simulink model "Simulation_6DOFTesting"  (R2024a)
settings: Solver=ode4  StartTime=initial_time  StopTime=final_time  FixedStep=timestep  RelTol=1e-3
values from neighbouring files (symbols this model uses):
  aEarth = 0    [CodeTesting_6DOF.m]    (also in Constants_6DOF.m = 6378137; Constants_6DOFTesting.m = 6378137)
  alphaArray = [-30, -25, -20, -15, -10, -5, 0, 5, 10, 15, 20, 25, 30]    [CodeTesting_6DOF.m]    (also in Constants_6DOF.m; Constants_6DOFTesting.m)
  altitudeArray = [0, 1000, 2000, 3000, 4000, 5000, 6000, 7000, 8000, 9000, 10000, 15000, 20000,      25000, 30000, 35000, 40000, 45000, 50000, 55000, 60000]    [CodeTesting_6DOF.m]    (also in Constants_6DOF.m; Constants_6DOFTesting.m)
  bEarth = 0    [CodeTesting_6DOF.m]    (also in Constants_6DOF.m = 6356752.3; Constants_6DOFTesting.m = 6356752.3)
  cD_3DArray = zeros(numAoAs, numMachs, numAltitudes)    [CodeTesting_6DOF.m]    (also in Constants_6DOF.m; Constants_6DOFTesting.m)
  cL_3DArray = zeros(numAoAs, numMachs, numAltitudes)    [CodeTesting_6DOF.m]    (also in Constants_6DOF.m; Constants_6DOFTesting.m)
  densityList = rhoList    [CodeTesting_6DOF.m]    (also in Constants_6DOF.m = usAtmosphere.x_; Constants_6DOFTesting.m = usAtmosphere.x_)
  height0 = 0    [Constants_6DOF.m]    (also in Constants_6DOFTesting.m = 5000)
  heightsList = usAtmosphere.Z    [CodeTesting_6DOF.m]    (also in Constants_6DOF.m; Constants_6DOFTesting.m)
  inertialPitch0 = deg2rad(inertialPitch0)    [Constants_6DOFTesting.m]
  inertialRoll0 = deg2rad(inertialRoll0)    [Constants_6DOFTesting.m]
  inertialYaw0 = deg2rad(inertialYaw0)    [Constants_6DOFTesting.m]
  Ixx = 10    [CodeTesting_6DOF.m]    (also in Constants_6DOF.m; Constants_6DOFTesting.m = 4.88094462)
  Ixz = 10    [CodeTesting_6DOF.m]    (also in Constants_6DOF.m = 1; Constants_6DOFTesting.m = 4.88094462)
  Iyy = 10    [CodeTesting_6DOF.m]    (also in Constants_6DOF.m; Constants_6DOFTesting.m = 4.88094462)
  Izz = 10    [CodeTesting_6DOF.m]    (also in Constants_6DOF.m; Constants_6DOFTesting.m = 4.88094462)
  latitude0 = pi/4    (= 0.785398163397)    [CodeTesting_6DOF.m]    (also in Constants_6DOF.m = deg2rad(latitude0); Constants_6DOFTesting.m = deg2rad(latitude0))
  longitude0 = pi/4    (= 0.785398163397)    [CodeTesting_6DOF.m]    (also in Constants_6DOF.m = deg2rad(longitude0); Constants_6DOFTesting.m = deg2rad(longitude0))
  m0 = 10    [CodeTesting_6DOF.m]    (also in Constants_6DOF.m = 50; Constants_6DOFTesting.m = 14.5939029)
  machArray = [0.5, 1.0, 1.5, 2.0, 2.5, 3.0, 3.5, 4.0, 4.5, 5.0, 5.5, 6.0, 6.5, 7.0, 7.5, 8.0,      8.5, 9.0, 9.5, 10.0]    [CodeTesting_6DOF.m]    (also in Constants_6DOF.m; Constants_6DOFTesting.m)
  omegaEarth = omega_earth    (= 7.2921159e-05)    [CodeTesting_6DOF.m]    (also in Constants_6DOF.m; Constants_6DOFTesting.m)
  p0Body = deg2rad(p0Body)    [Constants_6DOFTesting.m]
  phiBody0 = deg2rad(phiBody0)    [Constants_6DOFTesting.m]
  psiBody0 = deg2rad(psiBody0)    [Constants_6DOFTesting.m]
  q0Body = deg2rad(q0Body)    [Constants_6DOFTesting.m]
  r0Body = deg2rad(r0Body)    [Constants_6DOFTesting.m]
  rEarth = r_earth    (= 6371008.8)    [CodeTesting_6DOF.m]    (also in Constants_6DOF.m; Constants_6DOFTesting.m)
  temperatureList = usAtmosphere.T    [CodeTesting_6DOF.m]    (also in Constants_6DOF.m; Constants_6DOFTesting.m)
  thetaBody0 = deg2rad(thetaBody0)    [Constants_6DOFTesting.m]
  u0Body = 304.8    [Constants_6DOFTesting.m]
  v0Body = 0    [Constants_6DOFTesting.m]
  w0Body = -1 * w0Body    (= 0)    [Constants_6DOFTesting.m]
  wingArea = 0    [CodeTesting_6DOF.m]    (also in Constants_6DOF.m = 50; Constants_6DOFTesting.m = 0.09290304)
undefined symbols (not defined in the file or in its folder): inertialX0, inertialY0, inertialZ0
libraries: simulink_extras x18
(part 2 of 2)

== matlab function Simulation_6DOFTesting/Equations of Motion/Subsystem2/MATLAB Function1 ==
  data: r input; y output; q input; phi input
function y = fcn(r, q, phi)

y = q * cos(phi) - r * sin(phi);

== matlab function Simulation_6DOFTesting/Equations of Motion/Subsystem2/MATLAB Function2 ==
  data: r input; y output; q input; phi input; theta input
function y = fcn(r, q, phi, theta)

y = q * sin(phi) * sec(theta) + r * cos(phi) * sec(theta);

== matlab function Simulation_6DOFTesting/Control Surfaces/sideslipAngle ==
  data: t input; y output
function y = fcn(t)

sideslipAngle = 0;

y = sideslipAngle;

== matlab function Simulation_6DOFTesting/Equations of Motion/Subsystem2/MATLAB Function3 ==
  data: omegaEarth input; y output; latitude input; longitude input; positionNED input
function y = fcn(omegaEarth, latitude, longitude, positionNED)

omegaEarth = [0; 0; omegaEarth];

rotationMatrix = [(-1 * sin(latitude) * cos(longitude)) (-1 * sin(latitude) * sin(longitude)) (cos(latitude)); (-1 * sin(longitude)) (cos(longitude)) (0); (-1 * cos(latitude) * cos(longitude)) (-1 * cos(latitude) * sin(longitude)) (-1 * sin(latitude))];


velocityNEDFrame = rotationMatrix * omegaEarth;
positionNED = positionNED;

velocityRotatingEarth = cross(velocityNEDFrame, positionNED);


y = velocityRotatingEarth;

== matlab function Simulation_6DOFTesting/Equations of Motion/Subsystem2/MATLAB Function4 ==
  data: velocityRotatingEarth input; y output
function y = fcn(velocityRotatingEarth)

magnitudeRotatingEarth = norm(velocityRotatingEarth);

y = magnitudeRotatingEarth;

== matlab function Simulation_6DOFTesting/Coordinate Transformations/MATLAB Function ==
  data: positionNED input; y output; latitude input; longitude input
function y = fcn(positionNED, latitude, longitude)

rotationY = roty(pi/2 + latitude);
rotationZ = rotz(-1 * longitude);

rotationMatrix = rotationZ * rotationY;

cartesianECEF = rotationMatrix * positionNED;

y = cartesianECEF;

== matlab function Simulation_6DOFTesting/Coordinate Transformations/Polar ECEF - lat, long, height/MATLAB Function1 ==
  data: latitude input; longitude input; positionNED input; y output; latitude0 input; longitude0 input; height0 input; a input; b input; t input
function y = fcn( latitude, longitude, positionNED, latitude0, longitude0, height0, a, b, t)

rEarth = 6371.0088 * 10^3; 

long = longitude;
lat = latitude;

row1 = [-cos(long) * sin(lat) -sin(long) -cos(lat) * cos(long)];
row2 = [-sin(lat) * sin(long) cos(long) -cos(lat) * sin(long)];
row3 = [cos(lat) 0 -sin(lat)];

rotationMatrix = [row1; row2; row3];

positionNED(3) = positionNED(3) - rEarth;

e = sqrt(1 - b^2/a^2);
N = a * (1 - e^2 * sin(latitude0)^2)^(-1/2);

initialECEFX = (height0 + N) * cos(latitude0) * cos(longitude0);
initialECEFY = (height0 + N) * cos(latitude0) * sin(longitude0);
initialECEFZ = (height0 + N * (1 - e^2)) * sin(latitude0);

initialECEFPosition = [initialECEFX; initialECEFY; initialECEFZ]


positionECEF = rotationMatrix * positionNED + initialECEFPosition;

y = positionECEF;

== matlab function Simulation_6DOFTesting/Coordinate Transformations/Polar ECEF - lat, long, height/MATLAB Function2 ==
  data: x input; y input; z input; y output; a input; b input; latitude0 input
function y = fcn(x, y, z, a, b, latitude0)

   zLat = z
   r = sqrt(x^2 + y^2 + z^2)
   s = z/r
   c = sqrt(x^2 + y^2) / r
   e = sqrt(1 - b^2/a^2)
   a1 = a * e^2
   a2 = a^2 * e^4
   a3 = a * e^4 / 2
   a4 = (5/2) * a^2 * e^4

   factor1 = a1 + a2/r
   factor2 = s^2 * (a3 - a4/r)

   numerator = factor1 - factor2
   s1 = s * (1 + c^2 * (numerator / r))

   lambdaPrime = acos(z/r) * 180 / pi;

   testValue = 1 * 10^(-10);

    if x < testValue && x > -testValue
        x = 0.000001;
    end

    if y < testValue && y > -testValue
        y = 0.000001;
    end

   if lambdaPrime < 57

       lambda1 = asin(s1);
       a5 = a1 + a3 * lambda1;

   else

       c1 = sqrt(1 - s1^2);
       lambda1 = acos(c1);
       a5 = a1 + a3 * lambda1;

   end

    factor1 = a5 - a2/r;
    factor2 = c^2 * (a3 - a4/r);
    
    numerator = factor1 - factor2;

   c1 = c * (1 - s^2 * (numerator/r));

   fraction = a / sqrt(1 - e^2 * s1^2);
   product1 = s1 * (1 - e^2) * fraction;
   product2 = c1 * fraction;

   num = a * (1 - e^2);
   denum = (1 - e^2 * s1^2)^(3/2);

   m = c1 * ( z - product1 ) - s1 * ( sqrt(x^2 + y^2) - product2 );
   rC = (num / denum) + c1 * ( sqrt(x^2 + y^2) - product2 ) + s1 * ( z - product1 );

   latitude = lambda1 + m / rC;

   testLat = latitude * 180/pi
  


y = latitude;

== matlab function Simulation_6DOFTesting/Control Surfaces/AoA ==
  data: t input; y output
function y = fcn(t)

AoA = 0;

y = AoA;

== matlab function Simulation_6DOFTesting/Coordinate Transformations/Polar ECEF - lat, long, height/MATLAB Function3 ==
  data: x input; y input; y output; longitude0 input
function y = fcn(x, y, longitude0)

x = x;
y = y;


testValue = 1 * 10^(-10);

if x < testValue && x > -testValue
    x = 0.000001;
end

if y < testValue && y > -testValue
    y = 0.000001;
end

longitude =  atan2(y,x) + longitude0;


y = longitude;

== matlab function Simulation_6DOFTesting/Coordinate Transformations/Cartesian ECEF - x, y, z/MATLAB Function4 ==
  data: positionECEF input; y output
function y = fcn(positionECEF)

rEarth = 6371.0088 * 10^3;

height = norm(positionECEF) - rEarth;

y = height;

== matlab function Simulation_6DOFTesting/Coordinate Transformations/Polar ECEF - lat, long, height/MATLAB Function ==
  data: u input; y output
function y = fcn(u)

y = norm(u);

== matlab function Simulation_6DOFTesting/Coordinate Transformations/Cartesian ECEF - x, y, z/MATLAB Function ==
  data: u input; y output
function y = fcn(u)

y = norm(u);

== matlab function Simulation_6DOFTesting/Control Surfaces/rollSurfaceDeflection ==
  data: t input; y output
function y = fcn(t)

rollSurfaceDeflection = 0.0;

y = rollSurfaceDeflection;

== matlab function Simulation_6DOFTesting/Forces, Moments & their Coefficients/LiftZ ==
  data: rho input; y output; cl input; A input; v input
function y = fcn(rho, cl, A, v)

y = 0.5 * rho * v^2 * A * cl;

== matlab function Simulation_6DOFTesting/Forces, Moments & their Coefficients/DragX ==
  data: rho input; y output; v input; cd input; A input
function y = fcn(rho, v, cd, A)

Drag = 0.5 * rho * v^2 * A * cd;

y = Drag;

== matlab function Simulation_6DOFTesting/Atmospheric Conditions/g ==
  data: y output; r input
function y = fcn(r)

mu_earth = 3.986004418 * 10^14;
rE = 6378140;

y = mu_earth / (rE + r)^2;

== matlab function Simulation_6DOFTesting/Atmospheric Conditions/rho ==
  data: rhoList input; hList input; r input; y output
function y = fcn(rhoList, hList, r)

r = r / 10^3;

if r >= 0
    density = interp1(hList, rhoList, r);
else
    density = 0;
end


y = density;
